simulink model "agent_simulink"  (R2021b)
settings: Solver=VariableStepAuto  StartTime=0.0  StopTime=10.0  RelTol=1e-3
undefined symbols (not defined in the file): chargingStations
libraries: dspindex x1
settings Model: Creator=yekin  LastModifiedBy=yekin

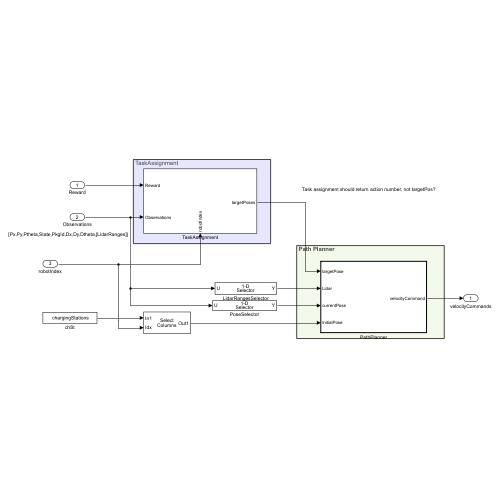
[thumbnail: Simulink's stored preview of the top-level diagram]
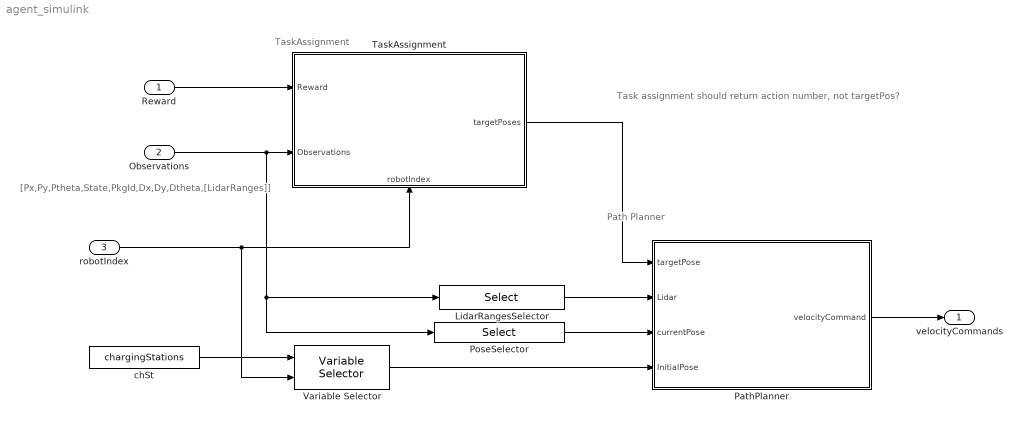
== system agent_simulink ==
  note: Path Planner
  note: TaskAssignment
  note: Task assignment should return action number, not targetPos?
  note: [Px,Py,Ptheta,State,PkgId,Dx,Dy,Dtheta,[LidarRanges]]
  Reward : Inport
  Observations : Inport  Port=2
  robotIndex : Inport  Port=3
  LidarRangesSelector : Selector  InputPortWidth=observationsLength  IndexOptions=Index vector (dialog)  Indices=lidarRangesIndex  OutputSizes=1
  PathPlanner : Subsystem  TreatAsAtomicUnit=on
  PoseSelector : Selector  InputPortWidth=observationsLength  IndexOptions=Index vector (dialog)  Indices=observationsLength  OutputSizes=1
  TaskAssignment : Subsystem
      settings: PortSchema="{\"entries\":[{\"content\":{\"sides\":[{\"content\":{\"connectorIds\":[\"In1\",\"In2\"]},\"type\":\"ConnectorPlacement.EquallySpacedRectSide\",\"uuid\":\"9c78a5d5-6efa-4587-a707-e931fe8561f2\"},{\"content\":{\"connectorIds\":[\"Out1\"],\"side\":\"RIGHT\"},\"type\":\"ConnectorPlacement.EquallySpacedRectSide\",\"uuid\":\"c290d152-0676-482f-a96f-0c7e79bd53cf\"},{\"content\":{\"connectorIds\":[],\"side\":\"TOP\"},\"type\":\"ConnectorPlacement.EquallySpacedRectSide\",\"uuid\":\"1da81dc1-8ac7-4dd7-afb8-538df59dce68\"},{\"content\":{\"connectorIds\":[\"In3\"],\"side\":\"BOTTOM\"},\"type\":\"ConnectorPlacement.EquallySpacedRectSide\",\"uuid\":\"d162df74-c928-426f-92ee-849b19f35adc\"}]},\"type\":\"ConnectorPlacement.EquallySpacedConnector\",\"uuid\":\"2fd73ab6-6cd9-46fb-a80a-c713a2435a49\"}],\"packageUris\":[\"http://schema.mathworks.com/mf0/Connector/R2020b\"],\"version\":\"1.0\"}"
  Variable Selector : dspindex/Variable Selector  NumInputs=1  rowsOrCols=Columns  IdxMode=Variable  Elements=[1 3]  ZerOneIdxMode=One-based  errmode=Clip Index  FillMode=on  FillValues=0
  chSt : Constant  Value=chargingStations
  velocityCommands : Outport
  wires:
  Variable Selector/1 -> PathPlanner/4(InitialPose)
  robotIndex/1 -> TaskAssignment/3(robotIndex), Variable Selector/2
  Reward/1 -> TaskAssignment/1(Reward)
  TaskAssignment/1(targetPoses) -> PathPlanner/1(targetPose)
  chSt/1 -> Variable Selector/1
  PoseSelector/1 -> PathPlanner/3(currentPose)
  Observations/1 -> PoseSelector/1, LidarRangesSelector/1, TaskAssignment/2(Observations)
  LidarRangesSelector/1 -> PathPlanner/2(Lidar)
  PathPlanner/1(velocityCommand) -> velocityCommands/1

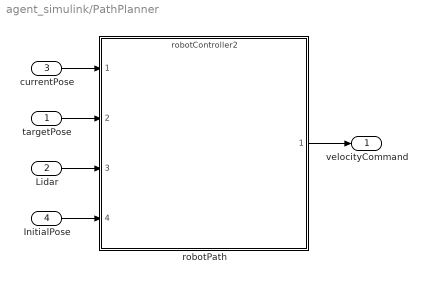
== system agent_simulink/PathPlanner ==
  targetPose : Inport
  Lidar : Inport  Port=2
  currentPose : Inport  Port=3
  InitialPose : Inport  Port=4
  robotPath : ModelReference  ModelNameDialog=robotController2.slx  ModelReferenceVersion=1.42
  velocityCommand : Outport
  wires:
  robotPath/1 -> velocityCommand/1
  currentPose/1 -> robotPath/1
  targetPose/1 -> robotPath/2
  Lidar/1 -> robotPath/3
  InitialPose/1 -> robotPath/4

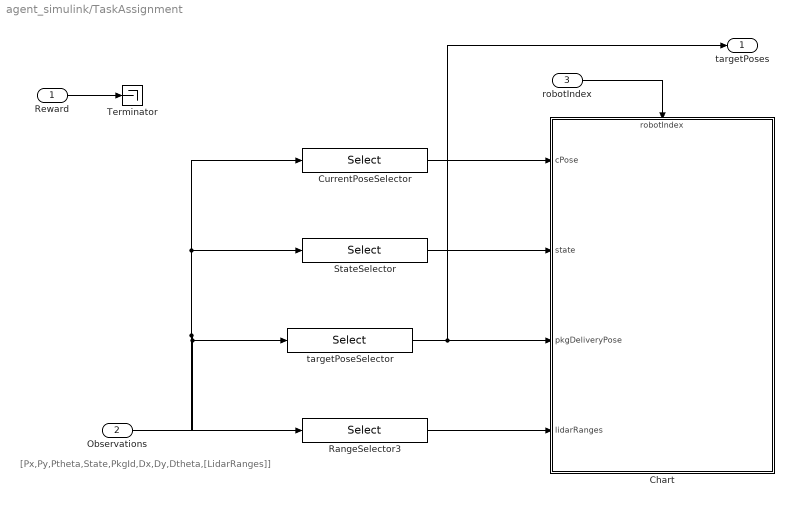
== system agent_simulink/TaskAssignment ==
  note: [Px,Py,Ptheta,State,PkgId,Dx,Dy,Dtheta,[LidarRanges]]
  Reward : Inport
  Observations : Inport  Port=2
  robotIndex : Inport  Port=3
  Chart : Stateflow chart  TreatAsAtomicUnit=on
      settings: PortSchema="{\"entries\":[{\"content\":{\"sides\":[{\"content\":{\"connectorIds\":[\"In2\",\"In3\",\"In4\",\"In5\"]},\"type\":\"ConnectorPlacement.EquallySpacedRectSide\",\"uuid\":\"443946ab-69a1-4568-8562-4e4f08676f63\"},{\"content\":{\"connectorIds\":[],\"side\":\"RIGHT\"},\"type\":\"ConnectorPlacement.EquallySpacedRectSide\",\"uuid\":\"6b1837f4-da10-47ca-91d1-5fafca2cde3a\"},{\"content\":{\"connectorIds\":[\"In1\"],\"side\":\"TOP\"},\"type\":\"ConnectorPlacement.EquallySpacedRectSide\",\"uuid\":\"64eea770-05bb-47ef-a9c1-8ed99a2aac36\"}]},\"type\":\"ConnectorPlacement.EquallySpacedConnector\",\"uuid\":\"82813f46-d2e1-4e6c-9c42-bee8482f8cb9\"}],\"packageUris\":[\"http://schema.mathworks.com/mf0/Connector/R2020b\"],\"version\":\"1.0\"}"
  CurrentPoseSelector : Selector  InputPortWidth=observationsLength  IndexOptions=Index vector (dialog)  Indices=ObsCurrendPoseIndexes  OutputSizes=1
  RangeSelector3 : Selector  InputPortWidth=observationsLength  IndexOptions=Index vector (dialog)  Indices=lidarRangesIndex  OutputSizes=1
  StateSelector : Selector  InputPortWidth=observationsLength  IndexOptions=Index vector (dialog)  Indices=stateIndex  OutputSizes=1
  Terminator : Terminator
  targetPoseSelector : Selector  InputPortWidth=observationsLength  IndexOptions=Index vector (dialog)  Indices=targetPosIndexes  OutputSizes=1
  targetPoses : Outport
  wires:
  Reward/1 -> Terminator/1
  CurrentPoseSelector/1 -> Chart/2(cPose)
  Observations/1 -> CurrentPoseSelector/1, StateSelector/1, RangeSelector3/1, targetPoseSelector/1
  StateSelector/1 -> Chart/3(state)
  targetPoseSelector/1 -> targetPoses/1, Chart/4(pkgDeliveryPose)
  RangeSelector3/1 -> Chart/5(lidarRanges)
  robotIndex/1 -> Chart/1(robotIndex)

== stateflow chart agent_simulink/TaskAssignment/Chart ==
  data: robotIndex input; cPose input; state input; pkgDeliveryPose input; lidarRanges input
